simulink model "exercise2"  (Simulink 7.1)
settings: Solver=ode45  StartTime=0.0  StopTime=1.0  RelTol=1e-3
settings Model: Creator=minyan09  LastModifiedBy=minyan09
settings DataIOCC: SaveOutput=off  SaveState=on

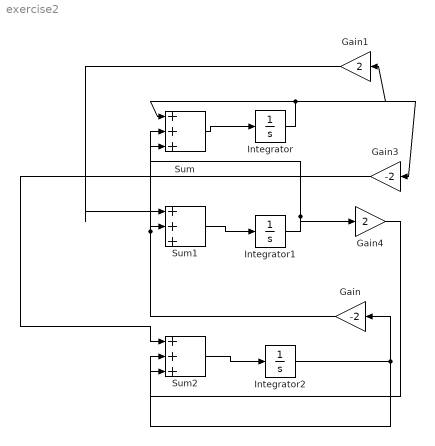
== system exercise2 ==
  Gain : Gain  Orientation=left  Gain=-2  ParameterDataType=sfix(16)  ParameterScaling=2^0  OutDataType=sfix(16)  OutScaling=2^0
  Gain1 : Gain  Orientation=left  Gain=2  ParameterDataType=sfix(16)  ParameterScaling=2^0  OutDataType=sfix(16)  OutScaling=2^0
  Gain3 : Gain  Orientation=left  Gain=-2  ParameterDataType=sfix(16)  ParameterScaling=2^0  OutDataType=sfix(16)  OutScaling=2^0
  Gain4 : Gain  Gain=2  ParameterDataType=sfix(16)  ParameterScaling=2^0  OutDataType=sfix(16)  OutScaling=2^0
  Integrator : Integrator  InitialCondition=2
  Integrator1 : Integrator  InitialCondition=1
  Integrator2 : Integrator  InitialCondition=1
  Sum : Sum  Inputs=|+++  OutDataType=sfix(16)  OutScaling=2^0
  Sum1 : Sum  Inputs=|+++  OutDataType=sfix(16)  OutScaling=2^0
  Sum2 : Sum  Inputs=|+++  OutDataType=sfix(16)  OutScaling=2^0
  wires:
  Sum/1 -> Integrator/1
  Integrator/1 -> Sum/1, Gain1/1, Gain3/1
  Integrator1/1 -> Sum/2, Gain4/1
  Integrator2/1 -> Gain/1, Sum2/3
  Gain/1 -> Sum/3, Sum1/2
  Gain1/1 -> Sum1/1
  Gain3/1 -> Sum2/1
  Gain4/1 -> Sum2/2
  Sum2/1 -> Integrator2/1
  Sum1/1 -> Integrator1/1
